simulink model "probm9"  (R2020a)
settings: Solver=ode45  StartTime=0.0  StopTime=30  MaxStep=0.01  RelTol=1e-3
model workspace (MAT data in the model file):
  B = Simulink.Parameter
  B.Value = 1e-06
  B.DataType = 'auto'
  B.Dimensions = [1 1]
  J = Simulink.Parameter
  J.Value = 1.517e-05
  J.DataType = 'auto'
  J.Dimensions = [1 1]
  Kw = Simulink.Parameter
  Kw.Value = 5.623e-05
  Kw.DataType = 'auto'
  Kw.Dimensions = [1 1]
  L = Simulink.Parameter
  L.Value = 0.00505
  L.DataType = 'auto'
  L.Dimensions = [1 1]
  P = Simulink.Parameter
  P.Value = 4
  P.DataType = 'auto'
  P.Dimensions = [1 1]
  R = Simulink.Parameter
  R.Value = 4.98
  R.DataType = 'auto'
  R.Dimensions = [1 1]
  Tl = Simulink.Parameter
  Tl.Value = 0.1
  Tl.DataType = 'auto'
  Tl.Dimensions = [1 1]
settings Model: ParameterArgumentNames=P  OrderedModelArguments=off  Creator=DELL  LastModifiedBy=DELL

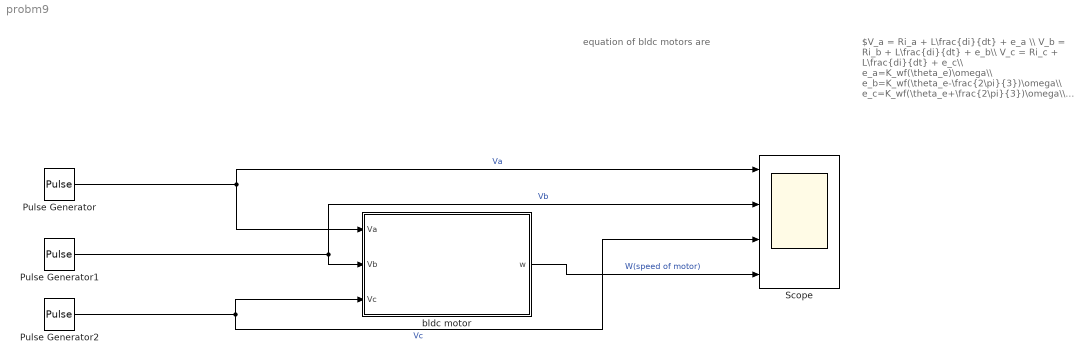
== system probm9 ==
  note: equation of bldc motors are
  note: $V_a = Ri_a + L\frac{di}{dt} + e_a \\ V_b = Ri_b + L\frac{di}{dt} + e_b\\ V_c = Ri_c + L\frac{di}{dt} + e_c\\ e_a=K_wf(\theta_e)\omega\\ e_b=K_wf(\theta_e-\frac{2\pi}{3})\omega\\ e_c=K_wf(\theta_e+\frac{2\pi}{3})\omega\\ \theta_e=\frac{P}{2}\theta_m\\ T_e=\frac{e_ai_b+e_bi_b+e_ci_c}{\omega}\\ T_e-T_l=J\frac{d\omega}{dt}+B\omega$
  Pulse Generator : DiscretePulseGenerator  PulseType=Time based  Amplitude=30  Period=10  PulseWidth=30
  Pulse Generator1 : DiscretePulseGenerator  PulseType=Time based  Amplitude=30  Period=10  PulseWidth=30  PhaseDelay=2.8
  Pulse Generator2 : DiscretePulseGenerator  PulseType=Time based  Amplitude=30  Period=10  PulseWidth=30  PhaseDelay=5.8
  Scope : Scope  NumInputPorts=4
  bldc motor : Subsystem
  wires:
  Pulse Generator/1 -> Scope/1, bldc motor/1(Va)  "Va"
  Pulse Generator1/1 -> Scope/2, bldc motor/2(Vb)  "Vb"
  Pulse Generator2/1 -> Scope/3, bldc motor/3(Vc)  "Vc"
  bldc motor/1(w) -> Scope/4  "W(speed of motor)"

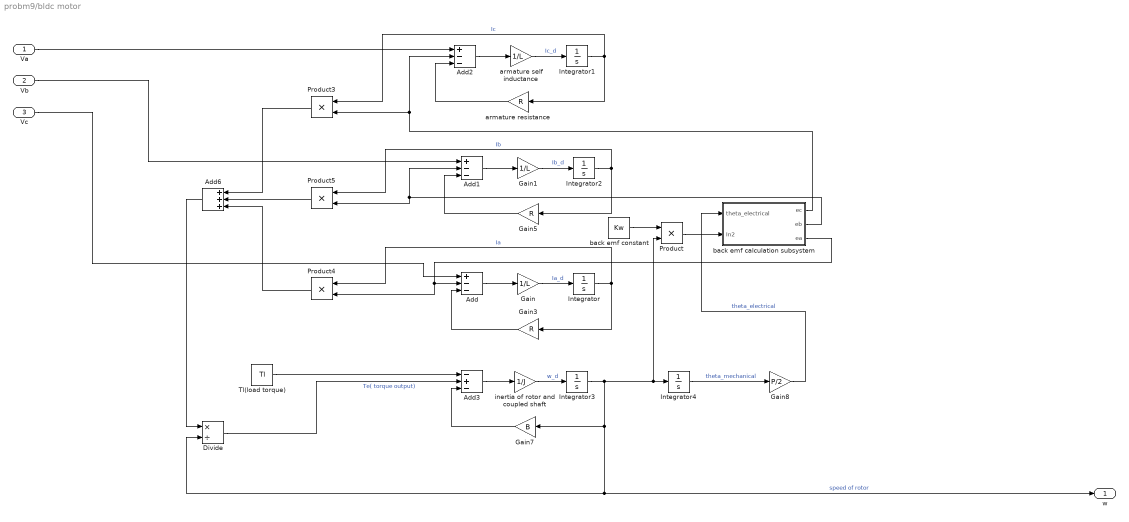
== system probm9/bldc motor ==
  Va : Inport
  Vb : Inport  Port=2
  Vc : Inport  Port=3
  Add : Sum  Inputs=+--
  Add1 : Sum  Inputs=+--
  Add2 : Sum  Inputs=+--
  Add3 : Sum  Inputs=-+-
  Add6 : Sum  Inputs=+++
  Divide : Product  Inputs=*/
  Gain : Gain  Gain=1/L
  Gain1 : Gain  Gain=1/L
  Gain3 : Gain  Gain=R
  Gain5 : Gain  Gain=R
  Gain7 : Gain  Gain=B
  Gain8 : Gain  Gain=P/2
  Integrator{,1..2,4} (4 alike) : Integrator
  Integrator3 : Integrator  InitialCondition=1
  Product{,3..5} (4 alike) : Product
  Tl(load torque) : Constant  Value=Tl
  armature resistance : Gain  Gain=R
  armature self inductance : Gain  Gain=1/L
  back emf calculation subsystem : Subsystem
  back emf constant : Constant  Value=Kw
  inertia of rotor and coupled shaft : Gain  Gain=1/J
  w : Outport
  wires:
  Product4/1 -> Add6/3
  Integrator3/1 -> Product/2, Integrator4/1, Gain7/1, w/1, Divide/2  "speed of rotor"
  Add1/1 -> Gain1/1
  Vc/1 -> Add/1
  Gain7/1 -> Add3/3
  Gain1/1 -> Integrator2/1  "Ib_d"
  Add3/1 -> inertia of rotor and coupled shaft/1
  Add2/1 -> armature self inductance/1
  Tl(load torque)/1 -> Add3/1
  inertia of rotor and coupled shaft/1 -> Integrator3/1  "w_d"
  armature self inductance/1 -> Integrator1/1  "Ic_d"
  Va/1 -> Add2/1
  Integrator/1 -> Gain3/1, Product4/1  "Ia"
  Integrator4/1 -> Gain8/1  "theta_mechanical"
  Vb/1 -> Add1/1
  Integrator2/1 -> Gain5/1, Product5/1  "Ib"
  Integrator1/1 -> armature resistance/1, Product3/1  "Ic"
  Gain3/1 -> Add/3
  Add6/1 -> Divide/1
  Product3/1 -> Add6/1
  Add/1 -> Gain/1
  Divide/1 -> Add3/2  "Te( torque output)"
  Gain/1 -> Integrator/1  "Ia_d"
  Product5/1 -> Add6/2
  Gain5/1 -> Add1/3
  armature resistance/1 -> Add2/3
  back emf calculation subsystem/2(eb) -> Add1/2, Product5/2
  back emf calculation subsystem/1(ec) -> Add2/2, Product3/2
  back emf calculation subsystem/3(ea) -> Product4/2, Add/2
  Gain8/1 -> back emf calculation subsystem/1(theta_electrical)  "theta_electrical"
  back emf constant/1 -> Product/1
  Product/1 -> back emf calculation subsystem/2(In2)

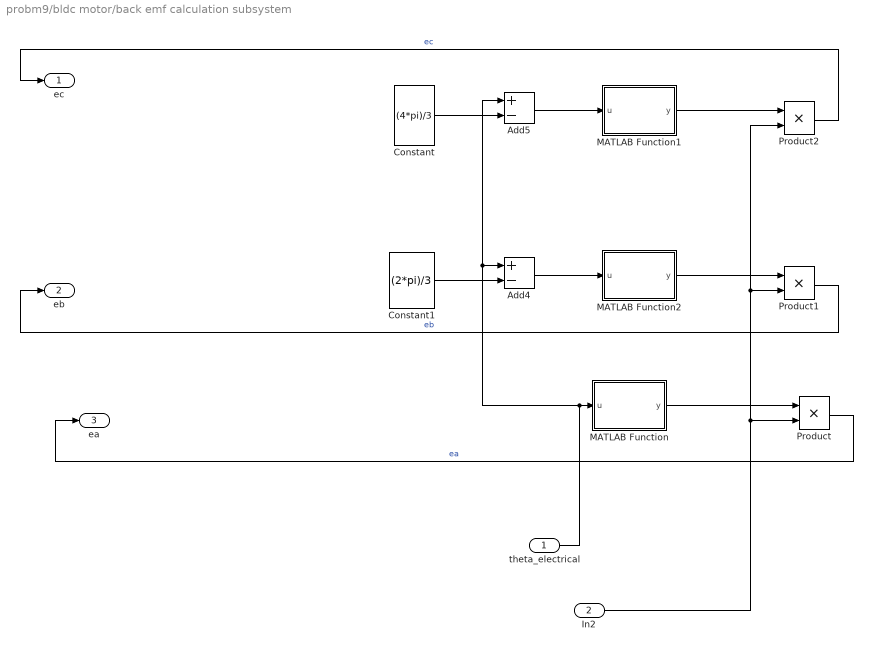
== system probm9/bldc motor/back emf calculation subsystem ==
  theta_electrical : Inport
  In2 : Inport  Port=2
  Add4 : Sum  Inputs=+-
  Add5 : Sum  Inputs=+-
  Constant : Constant  Value=(4*pi)/3
  Constant1 : Constant  Value=(2*pi)/3
  MATLAB Function : MATLAB Function  TreatAsAtomicUnit=on
  MATLAB Function1 : MATLAB Function  TreatAsAtomicUnit=on
  MATLAB Function2 : MATLAB Function  TreatAsAtomicUnit=on
  Product : Product
  Product1 : Product
  Product2 : Product
  ec : Outport
  eb : Outport  Port=2
  ea : Outport  Port=3
  wires:
  In2/1 -> Product2/2, Product1/2, Product/2
  theta_electrical/1 -> Add5/1, Add4/1, MATLAB Function/1(u)
  MATLAB Function/1(y) -> Product/1
  Add5/1 -> MATLAB Function1/1(u)
  MATLAB Function1/1(y) -> Product2/1
  Constant/1 -> Add5/2
  Add4/1 -> MATLAB Function2/1(u)
  Constant1/1 -> Add4/2
  MATLAB Function2/1(y) -> Product1/1
  Product1/1 -> eb/1  "eb"
  Product2/1 -> ec/1  "ec"
  Product/1 -> ea/1  "ea"

== matlab function probm9/bldc motor/back emf calculation subsystem/MATLAB Function ==
  data: u input; y output
function y = fcn(u)

if (u>=0 && u<((2*pi)/3))
    y = 1;
elseif(u>=((2*pi)/3) && u<pi)
    y = 1-(6/pi*(u-((2*pi)/3)));
elseif(u>=pi && u<((5*pi)/3))
    y = -1;
else
    y = -1+(6/pi*(u-((5*pi)/3)));
end
end

== matlab function probm9/bldc motor/back emf calculation subsystem/MATLAB Function2 ==
  data: u input; y output
function y = fcn(u)

if (u>=0 && u<((2*pi)/3))
    y = 1;
elseif(u>=((2*pi)/3) && u<pi)
    y = 1-(6/pi*(u-((2*pi)/3)));
elseif(u>=pi && u<((5*pi)/3))
    y = -1;
else
    y = -1+(6/pi*(u-((5*pi)/3)));
end
end

== matlab function probm9/bldc motor/back emf calculation subsystem/MATLAB Function1 ==
  data: u input; y output
function y = fcn(u)

if (u>=0 && u<((2*pi)/3))
    y = 1;
elseif(u>=((2*pi)/3) && u<pi)
    y = 1-(6/pi*(u-((2*pi)/3)));
elseif(u>=pi && u<((5*pi)/3))
    y = -1;
else
    y = -1+(6/pi*(u-((5*pi)/3)));
end
end
